simulink model "destilador_10c_sim_dos"  (R2018b)
settings: Solver=VariableStepAuto  StartTime=0.0  StopTime=17290  FixedStep=1  MaxStep=10  RelTol=1e-4  AbsTol=1e-5  EnableMultiTasking=on
InitFcn:
  | %% Condiciones iniciales
  | load('X0_ini_ev') %% 6/7/2018 20:06 cond_inicialx0.m % Cmet=1.5; % V=40; % GA=13; % N=21;
  | 
  | % Parameters
  | Mcp_c=4*50000;
  | Phi_ef=0.99;
  | V_m=20;  %mL volumen
  | Q_loss=0; % watt
  | GLm_0=80;
  | 
  | alpha=0.009;
  | F_fin=150;
  | F_ini=50;
  | 
  | 
  | %% Setting initial condition vector
  | x0_ini2=x0_ini;
  | N=7;
  | x0_ini=zeros(4*N+7,1);
  | x0_ini(1)=x0_ini2(1);
  | x0_ini(2)=x0_ini2(2);
  | x0_ini(3)=x0_ini2(3);
  | for J=1:N
  |   x0_ini(4*J+0)=(x0_ini2(4*J+0+8*(J-1))+x0_ini2(4*J+4+8*(J-1))+x0_ini2(4*J+8+8*(J-1)))/3;
  |   x0_ini(4*J+1)=(x0_ini2(4*J+1+8*(J-1))+x0_ini2(4*J+5+8*(J-1))+x0_ini2(4*J+9+8*(J-1)))/3+0.01;
  |   x0_ini(4*J+2)=(x0_ini2(4*J+2+8*(J-1))+x0_ini2(4*J+6+8*(J-1))+x0_ini2(4*J+10+8*(J-1)))/3;
  |   x0_ini(4*J+3)=(x0_ini2(4*J+3+8*(J-1))+x0_ini2(4*J+7+8*(J-1))+x0_ini2(4*J+11+8*(J-1)))/3;
  | end
  | 
  | b=2;
  | a=1;
  | x_min=[1767.71545621850;0.00799041062661984;3.41060000832915e-05;0.740207193810922;0.00799041062661984;3.41060000832915e-05;352.310691243690;0.740207193810922;0.00799041062661984;3.41060000832915e-05;352.310691243690;0.740207193810922;0.00799041062661984;3.41060000832915e-05;352.310691243690;0.740207193810922;0.00799041062661984;3.41060000832915e-05;352.310691243690;0.740207193810922;0.00799041062661984;3.41060000832915e-05;352.310691243690;0.740207193810922;0.00799041062661984;3.41060000832915e-05;352.310691243690;0.740207193810922;0.00799041062661984;3.41060000832915e-05;352.310691243690;0;0;0;0];
  | x_max=[2018.07587071285;0.624753322576231;0.000637824871562298;1.30537895369255;0.624753322576231;0.000637824871562298;371.461866693347;1.30537895369255;0.624753322576231;0.000637824871562298;371.461866693347;1.30537895369255;0.624753322576231;0.000637824871562298;371.461866693347;1.30537895369255;0.624753322576231;0.000637824871562298;371.461866693347;1.30537895369255;0.624753322576231;0.000637824871562298;371.461866693347;1.30537895369255;0.624753322576231;0.000637824871562298;371.461866693347;1.30537895369255;0.624753322576231;0.000637824871562298;371.461866693347;65.8799169826809;0.143158013086597;184.381691331991;91.0300185684774];
  | x_range=[250.360414494350;0.616762911949612;0.000603718871479006;0.565171759881627;0.616762911949612;0.000603718871479006;19.1511754496572;0.565171759881627;0.616762911949612;0.000603718871479006;19.1511754496572;0.565171759881627;0.616762911949612;0.000603718871479006;19.1511754496572;0.565171759881627;0.616762911949612;0.000603718871479006;19.1511754496572;0.565171759881627;0.616762911949612;0.000603718871479006;19.1511754496572;0.565171759881627;0.616762911949612;0.000603718871479006;19.1511754496572;0.565171759881627;0.616762911949612;0.000603718871479006;19.1511754496572;65.8799169826809;0.143158013086597;184.381691331991;91.0300185684774];
  | x_ss=0.5*(x_max+x_min);
  | 
  | 
  | No=7;  %ecuaciones externas BMyE columna
  | %Ajuste de estados auxiliares
  | x0_ini(4*N+3+1:4*N+No-1)=0;  % estados auxiliares
  | x0_ini(4*N+No)=GLm_0; % estado inicial de GLm
  | 
  | % int_lower_limit=[0 0 0, repmat([0 0 0 273+78],1,N),zeros(1,N-3)]';
  | % int_uper_limit=[5000 1 1, repmat([5 1 1 273+100],1,N),[5000 5000 5000 100]]';
  | 
  | 
  | 
  | 
  | %% Normalization values / mesurements
  | y_ss=76.5;
  | y_max=95;
  | y_min=30;
  | 
  | %% Normalization values / input/disturbances
  | u_ss=[1000 273+25 180];  % [Fr Qb Ti]
  | u_max=[1800 273+50 500];  % [Fr Qb Ti]
  | u_min=[100 273 5];  % [Fr Qb Ti]
values from neighbouring files (symbols this model uses):
  T_fin = dist_exp{i}(end,2)*60    [fcost.m]    (also in fcost_Fr.m; fcost_Fr2.m; fcost_Fr4.m; fcost_Fr5.m)
undefined symbols (not defined in the file or in its folder): Qb_0, Ti_0
libraries: simulink x1, jMPClib x1
(part 2 of 2)

== matlab function destilador_10c_sim_dos/NL Plant Nominal/Implicit Fun ==
  data: x input size=35; w input size=2; f output size=2; u input size=3; p input size=4
function f  = Implicit_fun(x,w,u,p)

Fr     = u(1);   % Flow refrigerant 
Tr     = u(2);   % Temperature refrigerant inlet
Qb     = u(3);   % Heating power boiler

x1c=w(1);  % implicit variable - liquid molar fraction ethanol condenser
Tout=w(2); % implicit variable - Temperature outlet coil condenser

phi_ef = p(1);

% phi_ef=0.701;


N=7;  % stages
No=7; % Aditional stat for output calculation
Ds = 2.047*2.54/100;                                                      % [m]
S = 0.25*pi*Ds^2;                                                   % [m^2]
ap = phi_ef*771; % Nominal, 0.83                                 % [m^2/m^3]                          
l = 0.25;                                                             % [m]
mr = 1933*5/8;                                                         % [g]                         
mrp = mr/l;                                                         % [g/m]
PM_EtOH = 46.07;                                                  % [g/mol]
PM_MetOH = 32.04;                                                 % [g/mol]
PM_H2O = 18.016;                                                  % [g/mol]
CM = 1.130;                                                           % [-]                                   
g = 9.8;                                                          % [m/s^2]
cpr = 0.474;                                                   % [J/(gr*K)]
Ta = 298.45;                                                          % [K]

z = linspace(0,l,N);
dz = z(2)-z(1);

% Luego se leen los estados con el fin de simplificarlo:
Mb = x(1);
x1b = x(2);
x2b = x(3);

M = zeros(1,N);
x1 = zeros(1,N);
x2 = zeros(1,N);
T = zeros(1,N);

for i = 1:N
    M(i) = x(4*i);
    x1(i) = x(4*i+1);
    x2(i) = x(4*i+2);
    T(i) = x(4*i+3);
end

GL_m    = x(4*N+No);  % Estado GL medido

% A continuación se presentan las ecuaciones algebraicas del modelo:
L= flujo_liquido2(M,x1,T,PM_EtOH,PM_H2O,g,ap,S); %vector flujo liquido
h = (55.678*x1+75.425).*T-15208.44*x1-20602.34; %vector de entalpía liquida

% Etapa 5: Presentaci?n de las propiedades del re-hervidor:
y1b = (1220*x1b^3-735.1*x1b^2+1220*x1b+1.498)/(x1b^3+54.93*x1b^2+1538*x1b+113);
Tb = (374.1+5855*x1b)/(1+16.65*x1b+0.1086*x1b^2);
y2b = equil2x(x1b,x2b,Tb);
hb = (55.678*x1b+75.425)*Tb-15208.44*x1b-20602.34;
Hb = 36172.03-2919.83*y1b+(31.461-11.976*y1b)*Tb+(4.063e-4+0.0734*y1b)*Tb^2;
dhbdx1b = 55.678*Tb-15208.44;
dhbdTb = 55.678*x1b+75.425;
dTbdx1b = (5855*(1+16.65*x1b+0.1086*x1b^2)-(374.1+5855*x1b)*(16.65+0.2172*x1b))/((1+16.65*x1b+0.1086*x1b)^2);
Qp = -190.45051+0.027736447*Tb^1.5-0.00069779137*Ta^2+(31705.067/Ta); % [W]
Qbe = Qb-Qp;                                                          % [W]
Vb = (L(1)*((h(1)-hb)+(dhbdx1b+dhbdTb*dTbdx1b)*(x1b-x1(1)))+Qbe)/((dhbdx1b+dhbdTb*dTbdx1b)*(x1b-y1b)+(Hb-hb));

% Etapa 6: C?lculo de las propiedades del vapor que pasa por la columna:
% - Etapa 1:
y1 = zeros(1,N);
y1_1=zeros(1,N);
y1_2=zeros(1,N);

% if T(1) <= 351.89
%     y1(1) = 0.5144798703316682*T(1)^2-362.04116781517121*T(1)+63693.126284857615;
% else if T(1) > 351.89 && T(1) < 362.15
%         y1(1) = -0.00029699079694785408*T(1)^3+0.31993865536139598*T(1)^2-114.90802529355385*T(1)+13759.682820348055;
%     else
%         y1(1) = -0.033707692307692737*T(1)+12.59634076923092;
%     end
% end


if T(1) <= 351.89
    y1(1) = 0.5144798703316682*T(1)^2-362.04116781517121*T(1)+63693.126284857615;
else %if T(1) > 351.89 && T(1) < 362.15
        y1_1(1) = -0.00029699079694785408*T(1)^3+0.31993865536139598*T(1)^2-114.90802529355385*T(1)+13759.682820348055;
%     else
        y1_2(1) = -0.033707692307692737*T(1)+12.59634076923092;
%     end
        sigma=1/(1+exp(-(T(1)-362.15)/1));
        y1(1)=(1-sigma)*y1_1(1)+sigma*y1_2(1);
end


% y1(1)=(1220*x1(1)^3-735.1*x1(1)^2+1220*x1(1)+1.498)/(x1(1)^3+54.93*x1(1)^2+1538*x1(1)+113);
% y1(1)=-3.103366261118440e-07*T(1)^7+ 7.760667779409546e-04*T(1)^6 -0.831728013863949*T(1)^5+ 4.952038647403622e+02*T(1)^4 -1.769012642424244e+05*T(1)^3+3.791596072579136e+07*T(1)^2 -4.514749479837228e+09*T(1)+ 2.303888385771235e+11;
% y1(1)=-1.836023738004047e-07*T(1)^7+ 4.634679433890438e-04*T(1)^6 -0.501379863593959*T(1)^5+ 3.013173444220613e+02*T(1)^4 -1.086463611148553e+05*T(1)^3+ 2.350390640205018e+07*T(1)^2 -2.824717157188236e+09*T(1)+ 1.454841438795462e+11;

    if y1(1)>.8947                                                 %límite azeótropo P atm.
        y1(1)=.8947;
    end

x1i = zeros(1,N);
x1i(1) = 1/(400*y1(1)^4-1299*y1(1)^3+1586*y1(1)^2-865*y1(1)+179.6);

% (PARENTESIS): Se construye un vector de par?metros que es necesario para
% poder llamar al macro transf_masa2:

param = [N PM_EtOH PM_H2O CM ap S g Qb dz 1 mrp cpr Ta]; % Unidades varias.

% Una vez hecho esto se inicializan las variables de flujo molar de vapor
% que sale de cada etapa, coeficientes de transferencia de masa, presi?n de
% vapor del metanol, coeficiente de actividad de ?ste en fase l?quida, u-
% tilizando el modelo de coeficiente de actividad NRTL. Adem?s se definen
% la fracci?n molar de metanol en el vapor y entalp?a de dicha fase,

k13aef = zeros(1,N);
V = zeros(1,N);
k21aef = zeros(1,N);
k23aef = zeros(1,N);
keqaef = zeros(1,N);
P2vap = zeros(1,N);
gama2 = zeros(1,N);
y2 = zeros(1,N);
H = zeros(1,N);

% (FIN DEL PARENTESIS)

Kaef = transf_masa2(x1(1),L(1),T(1),param);
k13aef(1) = Kaef(1,1);
V(1) = ((y1(1)*Vb/dz)+param(10)*S*k13aef(1)*(x1(1)-x1i(1)))/((2*y1(1)-y1b)/dz);
k21aef(1) = Kaef(1,2);
k23aef(1) = Kaef(1,3);
keqaef(1) = (k23aef(1)*k21aef(1)/(x1(1)*k23aef(1)+(1-x1(1))*k21aef(1)));
equil = equilibrio(x1i(1),T(1));
P2vap(1) = equil(1,1);
gama2(1) = equil(1,2);
y2(1) = ((V(1)*y2b/dz)+param(10)*S*keqaef(1)*x2(1))/(((2*V(1)-Vb)/dz)+(param(10)*S*keqaef(1)*101.325/(P2vap(1)*gama2(1))));
H(1) = 36172.03-2919.83*y1(1)+(31.461-11.976*y1(1))*T(1)+(4.063e-4+0.0734*y1(1))*T(1)^2;

% - Etapa 2 a N:
for i = 2:N
    
%     if T(i) <= 351.89
%         y1(i) = 0.5144798703316682*T(i)^2-362.04116781517121*T(i)+63693.126284857615;
%     else if T(i) > 351.89 && T(i) < 362.15
%             y1(i) = -0.00029699079694785408*T(i)^3+0.31993865536139598*T(i)^2-114.90802529355385*T(i)+13759.682820348055;
%         else
%             y1(i) = -0.033707692307692737*T(i)+12.59634076923092;
%         end
%         
%     end
%     
    if T(i) <= 351.89
        y1(i) = 0.5144798703316682*T(i)^2-362.04116781517121*T(i)+63693.126284857615;
    else %if T(i) > 351.89 && T(i) < 362.15
            y1_1(i) = -0.00029699079694785408*T(i)^3+0.31993865536139598*T(i)^2-114.90802529355385*T(i)+13759.682820348055;
%         else
            y1_2(i) = -0.033707692307692737*T(i)+12.59634076923092;
%         end
        sigma=1/(1+exp(-(T(i)-362.15)/1));
        y1(i)=(1-sigma)*y1_1(i)+sigma*y1_2(i);
    end
%     
% y1(i)=(1220*x1(i)^3-735.1*x1(i)^2+1220*x1(i)+1.498)/(x1(i)^3+54.93*x1(i)^2+1538*x1(i)+113);
% y1(i)=-3.103366261118440e-07*T(i)^7+ 7.760667779409546e-04*T(i)^6 -0.831728013863949*T(i)^5+ 4.952038647403622e+02*T(i)^4 -1.769012642424244e+05*T(i)^3+3.791596072579136e+07*T(i)^2 -4.514749479837228e+09*T(i)+ 2.303888385771235e+11;    
% y1(i)=-1.836023738004047e-07*T(i)^7+ 4.634679433890438e-04*T(i)^6 -0.501379863593959*T(i)^5+ 3.013173444220613e+02*T(i)^4 -1.086463611148553e+05*T(i)^3+ 2.350390640205018e+07*T(i)^2 -2.824717157188236e+09*T(i)+ 1.454841438795462e+11;
    if y1(i)>.8947                                                 %límite azeótropo P atm.
        y1(i)=.8947;
    end
    x1i(i) = 1/(400*y1(i)^4-1299*y1(i)^3+1586*y1(i)^2-865*y1(i)+179.6);
    Kaef = transf_masa2(x1(i),L(i),T(i),param);
    k13aef(i) = Kaef(1,1);
    V(i) = ((y1(i)*V(i-1)/dz)+param(10)*S*k13aef(i)*(x1(i)-x1i(i)))/((2*y1(i)-y1(i-1))/dz);
    k21aef(i) = Kaef(1,2);
    k23aef(i) = Kaef(1,3);
    keqaef(i) = (k23aef(i)*k21aef(i)/(x1(i)*k23aef(i)+(1-x1(i))*k21aef(i)));
    equil = equilibrio(x1i(i),T(i));
    P2vap(i) = equil(1,1);
    gama2(i) = equil(1,2);
    y2(i) = ((V(i)*y2(i-1)/dz)+param(10)*S*keqaef(i)*x2(i))/(((2*V(i)-V(i-1))/dz)+(param(10)*S*keqaef(i)*101.325/(P2vap(i)*gama2(i))));
    H(i) = 36172.03-2919.83*y1(i)+(31.461-11.976*y1(i))*T(i)+(4.063e-4+0.0734*y1(i))*T(i)^2;
end

%% Partial Condenser Column-side
% xc Implicit variable

%     T = (369.6-863.6*y1(N)+1049*y1(N)^2)/(1-2.34*y1(N)+2.918*y1(N)^2);                % [K]                 
    Hn = 36172.03-2919.83*y1(N)+(31.461-11.976*y1(N))*T(N)+(4.063e-4+0.0734*y1(N))*T(N)^2; % [J/mol]
    yD = (1220*x1c^3-735.1*x1c^2+1220*x1c+1.498)/(x1c^3+54.93*x1c^2+1538*x1c+113); % [-]
    R = (yD-y1(N))/(y1(N)-x1c);                                              % [-]
    Lc = V(N)/(1+(1/R));                                             % [mol/s]
    Tc = (374.1+5855*x1c)/(1+16.65*x1c+0.1086*x1c^2);                    % [K]
    equil = equilibrio(x1c,Tc);                          % [Unidades varias]                               
    P2vap = equil(1,1);                                             % [kPa]                                                
    gama2 = equil(1,2);                                               % [-]
    x2c = V(N)*y2(N)/(Lc*(1+(P2vap*gama2/(101.325*R))));                    % [-]
    hc = (55.678*x1c+75.425)*Tc-15208.44*x1c-20602.34;              % [J/mol]
    HD = 36172.03-2919.83*yD+(31.461-11.976*yD)*Tc+(4.063e-4+0.0734*yD)*Tc^2; % [J/mol]
    
    Qc_ef = V(N)*Hn-Lc*(hc+(HD/R));                                       % [W]


    
    
%% Partial Condenser Tube-side
% Tout  Implicit variable


T_film = 0.5*(Tr+Tout);                                              % [K]
cp = 0.000008935*T_film^2-0.0054919213*T_film+5.0225997509;   % [kJ/(kg*K)]
mu = exp((-9.108111-(753.33377/T_film)+(410019.22/(T_film^2))));   % [Pa*s]
k = -0.000008072*T_film^2+0.006348737*T_film-0.5649534949;      % [W/(m*K)]
Pr = exp((-8.9216883+0.00000062007495*T_film^2.5+(2915.8766/T_film))); % [-]

% ... y de la temperatura de la pared.

mu_s = exp((-9.108111-(753.33377/Tc)+(410019.22/(Tc^2))));         % [Pa*s]

% Ahora se procede a calcular las condiciones para el número de Nusselt, 
% antes se presentan los parámetros geométricos del serpentín:

As = 157.4776*(0.01^2);                                                  % [m^2]
do = 0.008;                                                           % [m]
di=0.007;
Long = As/(pi*do);                                                       % [m]

rho_def = -0.00295*(Tr)^2+1.45738*(Tr)+824.9622;

m = Fr*rho_def*(1/(60*1000*1000) );                                     % [kg/s]

Re = (4*m)/(pi*di*mu);                                                % [-]
Gz_mod = ((Re*Pr/(Long/do)))^(1/3)*((mu/mu_s))^(0.14);                   % [-]                                           
if (Re < 10000) && (Gz_mod < 2)
    Nu = 3.66;                                                        % [-]
else if (Re < 10000) && (Gz_mod >= 2)
       Nu = 1.86*Gz_mod;                                              % [-]
    else
        Nu = 0.027*Re^(4/5)*Pr^(1/3)*(mu/mu_s)^(0.14);                % [-]
    end
end

% Tras esto se calcula el coeficiente de transferencia de calor para el
% flujo refrigerante:

h_conv = k*Nu/do;                                                  % [W/(m^2*K)]

% Finalmente se calcula el largo del serpentín de dos formas independientes
% y se realiza la comparación entre ellos y la salida:

dTml = (Tout-Tr)/log((Tc-Tr)/(Tc-Tout))    ;                       % [K]
% dTml =(Tout*Tr*(Tr+Tc)/2)^(1/3);
Qc_I = h_conv*As*dTml;                                                     % [W]

 
cp_def = 0.000008935*(0.5*(Tr+Tout))^2-0.0054919213*(0.5*(Tr+Tout))+5.0225997509; % [kJ/(kg*K)]


Qc= Fr*(1/(60*1000)) * cp_def * (Tout-Tr) * rho_def;
    
% 
% destil = destilado(V(N),y1(N),y2(N),Lc,x1c,x2c,PM_EtOH,PM_H2O);
% GL=destil(1,1);
% Dvol=destil(1,2);
%     salida = [GL Dvol D_EtOH D_MEtOH D_H2O];  


f=zeros(2,1);
f(1)= (Qc-Qc_ef);  % Implicit equation 1
f(2)= (Qc-Qc_I);  % Implicit equation 2

== matlab function destilador_10c_sim_dos/NL Plant Nominal/ODE Distiller ==
  data: x input size=35; w input size=2; x_dot output size=35; u input size=3; y output size=12; p input size=4; x0 input size=35
function [x_dot,y] = ODE_Distiller(x,w,u,p,x0)
% Fr     = u(1);   % Flow refrigerant 
% Tr     = u(2);   % Temperature refrigerant inlet
Qb     = u(3);   % Heating power boiler

x1c=w(1);  % implicit variable - liquid molar fraction ethanol condenser
% Tout=w(2); % implicit variable - Temperature outlet coil condenser

phi_ef = p(1);
Mcp_c=p(2);
Q_loss=p(4);

N=7;  % stages
No=7; % Aditional stat for output calculation
Ds = 2.047*2.54/100;                                                      % [m]
S = 0.25*pi*Ds^2;                                                   % [m^2]
ap = phi_ef*771; % Nominal, 0.83                                 % [m^2/m^3]                          
l = 0.25;                                                             % [m]
mr = 1933*5/8;                                                         % [g]                         
mrp = mr/l;                                                         % [g/m]
PM_EtOH = 46.07;                                                  % [g/mol]
PM_MetOH = 32.04;                                                 % [g/mol]
PM_H2O = 18.016;                                                  % [g/mol]
CM = 1.130;                                                           % [-]                                   
g = 9.8;                                                          % [m/s^2]
cpr = 0.474;                                                   % [J/(gr*K)]
Ta = 298.45;                                                          % [K]

z = linspace(0,l,N);
dz = z(2)-z(1);

% Luego se leen los estados con el fin de simplificarlo:
Mb = x(1);
x1b = x(2);
x2b = x(3);

M =x(4+0:4:4*N+0);
x1=x(4+1:4:4*N+1);
x2=x(4+2:4:4*N+2);
T =x(4+3:4:4*N+3);

GL_m    = x(4*N+No);  % Estado GL medido

% A continuación se presentan las ecuaciones algebraicas del modelo:
L= flujo_liquido2(M,x1,T,PM_EtOH,PM_H2O,g,ap,S); %vector flujo liquido
h = (55.678*x1+75.425).*T-15208.44*x1-20602.34; %vector de entalpía liquida

% Etapa 5: Presentaci?n de las propiedades del re-hervidor:
coef_num_y_eq=[1220 -735.1 1220 1.498];
coef_den_y_eq=[1 54.93 1538 113];
y1b = polyval(coef_num_y_eq,x1b)/polyval(coef_den_y_eq,x1b);

Tb = (374.1+5855*x1b)/(1+16.65*x1b+0.1086*x1b^2);
y2b = equil2x(x1b,x2b,Tb);
hb = (55.678*x1b+75.425)*Tb-15208.44*x1b-20602.34;
Hb = 36172.03-2919.83*y1b+(31.461-11.976*y1b)*Tb+(4.063e-4+0.0734*y1b)*Tb^2;
dhbdx1b = 55.678*Tb-15208.44;
dhbdTb = 55.678*x1b+75.425;
dTbdx1b = (5855*(1+16.65*x1b+0.1086*x1b^2)-(374.1+5855*x1b)*(16.65+0.2172*x1b))/((1+16.65*x1b+0.1086*x1b)^2);
Qp = -190.45051+0.027736447*Tb^1.5-0.00069779137*Ta^2+(31705.067/Ta); % [W]
Qbe = Qb-Qp;                                                          % [W]
Vb = (L(1)*((h(1)-hb)+(dhbdx1b+dhbdTb*dTbdx1b)*(x1b-x1(1)))+Qbe)/((dhbdx1b+dhbdTb*dTbdx1b)*(x1b-y1b)+(Hb-hb));



y1_1 = -0.00029699079694785408*T.^3+0.31993865536139598*T.^2-114.90802529355385*T+13759.682820348055;
y1_2 = -0.033707692307692737*T+12.59634076923092;
sigma=1./(1+exp(-(T-362.15)/1));
y1=(1-sigma).*y1_1+sigma.*y1_2;


x1i = 1./(400*y1.^4-1299*y1.^3+1586*y1.^2-865*y1+179.6);

param = [N PM_EtOH PM_H2O CM ap S g Qb dz 1 mrp cpr Ta]; % Unidades varias.

% Una vez hecho esto se inicializan las variables de flujo molar de vapor
% que sale de cada etapa, coeficientes de transferencia de masa, presi?n de
% vapor del metanol, coeficiente de actividad de ?ste en fase l?quida, u-
% tilizando el modelo de coeficiente de actividad NRTL. Adem?s se definen
% la fracci?n molar de metanol en el vapor y entalp?a de dicha fase,

k13aef = zeros(1,N);
V = zeros(1,N);
k21aef = zeros(1,N);
k23aef = zeros(1,N);
keqaef = zeros(1,N);
P2vap = zeros(1,N);
gama2 = zeros(1,N);
y2 = zeros(1,N);
H = zeros(1,N);

% (FIN DEL PARENTESIS)

Kaef = transf_masa2(x1(1),L(1),T(1),param);
k13aef(1) = Kaef(1,1);
V(1) = ((y1(1)*Vb/dz)+param(10)*S*k13aef(1)*(x1(1)-x1i(1)))/((2*y1(1)-y1b)/dz);
k21aef(1) = Kaef(1,2);
k23aef(1) = Kaef(1,3);
keqaef(1) = (k23aef(1)*k21aef(1)/(x1(1)*k23aef(1)+(1-x1(1))*k21aef(1)));
equil = equilibrio(x1i(1),T(1));
P2vap(1) = equil(1,1);
gama2(1) = equil(1,2);
y2(1) = ((V(1)*y2b/dz)+param(10)*S*keqaef(1)*x2(1))/(((2*V(1)-Vb)/dz)+(param(10)*S*keqaef(1)*101.325/(P2vap(1)*gama2(1))));
H(1) = 36172.03-2919.83*y1(1)+(31.461-11.976*y1(1))*T(1)+(4.063e-4+0.0734*y1(1))*T(1)^2;


for i = 2:N
    Kaef = transf_masa2(x1(i),L(i),T(i),param);
    k13aef(i) = Kaef(1,1);
    V(i) = ((y1(i)*V(i-1)/dz)+param(10)*S*k13aef(i)*(x1(i)-x1i(i)))/((2*y1(i)-y1(i-1))/dz);
    k21aef(i) = Kaef(1,2);
    k23aef(i) = Kaef(1,3);
    keqaef(i) = (k23aef(i)*k21aef(i)/(x1(i)*k23aef(i)+(1-x1(i))*k21aef(i)));
    equil = equilibrio(x1i(i),T(i));
    P2vap(i) = equil(1,1);
    gama2(i) = equil(1,2);
    y2(i) = ((V(i)*y2(i-1)/dz)+param(10)*S*keqaef(i)*x2(i))/(((2*V(i)-V(i-1))/dz)+(param(10)*S*keqaef(i)*101.325/(P2vap(i)*gama2(i))));
    H(i) = 36172.03-2919.83*y1(i)+(31.461-11.976*y1(i))*T(i)+(4.063e-4+0.0734*y1(i))*T(i)^2;
end

    yD = polyval(coef_num_y_eq,x1c)/polyval(coef_den_y_eq,x1c);
    R = (yD-y1(N))/(y1(N)-x1c);                                              % [-]
    Lc = V(N)/(1+(1/R));                                             % [mol/s]
    Tc = (374.1+5855*x1c)/(1+16.65*x1c+0.1086*x1c^2);                    % [K]
    equil = equilibrio(x1c,Tc);                          % [Unidades varias]                               
    P2vap = equil(1,1);                                             % [kPa]                                                
    gama2 = equil(1,2);                                               % [-]
    x2c = V(N)*y2(N)/(Lc*(1+(P2vap*gama2/(101.325*R))));                    % [-]
    hc = (55.678*x1c+75.425)*Tc-15208.44*x1c-20602.34;              % [J/mol]

% Finalmente se presentan las ecuaciones diferenciales del modelo:
x_dot=zeros(4*N+No,1);

x_dot(1) = L(1)-Vb;
x_dot(2) = (1/Mb)*(L(1)*(x1(1)-x1b)-Vb*(y1b-x1b));
x_dot(3) = (1/Mb)*(L(1)*(x2(1)-x2b)-Vb*(y2b-x2b));
x_dot(4) = ((L(2)-L(1))/dz)+((Vb-V(1))/dz);
x_dot(5) = (1/M(1))*(L(1)*((x1(2)-x1(1))/dz)+V(1)*((y1b-y1(1))/dz)+(x1(1)-y1(1))*((V(1)-Vb)/dz));
x_dot(6) = (1/M(1))*(L(1)*((x2(2)-x2(1))/dz)+V(1)*((y2b-y2(1))/dz)+(x2(1)-y2(1))*((V(1)-Vb)/dz));
x_dot(7) = ((Mcp_c+mrp*cpr+M(1)*(55.678*x1(1)+75.425))^-1)*(-Q_loss/dz+L(1)*((h(2)-h(1))/dz)+V(1)*((Hb-H(1))/dz)+(h(1)-H(1))*((V(1)-Vb)/dz)-(55.678*T(1)-15208.44)*(L(1)*((x1(2)-x1(1))/dz)+V(1)*((y1b-y1(1))/dz)+(x1(1)-y1(1))*((V(1)-Vb)/dz)));
for i = 2:(N-1)
    x_dot(4*i) = ((L(i+1)-L(i))/dz)+((V(i-1)-V(i))/dz);
    x_dot(4*i+1) = (1/M(i))*(L(i)*((x1(i+1)-x1(i))/dz)+V(i)*((y1(i-1)-y1(i))/dz)+(x1(i)-y1(i))*((V(i)-V(i-1))/dz));
    x_dot(4*i+2) = (1/M(i))*(L(i)*((x2(i+1)-x2(i))/dz)+V(i)*((y2(i-1)-y2(i))/dz)+(x2(i)-y2(i))*((V(i)-V(i-1))/dz));
    x_dot(4*i+3) = ((Mcp_c+mrp*cpr+M(i)*(55.678*x1(i)+75.425))^-1)*(-Q_loss/dz+L(i)*((h(i+1)-h(i))/dz)+V(i)*((H(i-1)-H(i))/dz)+(h(i)-H(i))*((V(i)-V(i-1))/dz)-(55.678*T(i)-15208.44)*(L(i)*((x1(i+1)-x1(i))/dz)+V(i)*((y1(i-1)-y1(i))/dz)+(x1(i)-y1(i))*((V(i)-V(i-1))/dz)));
end
x_dot(4*N) = ((Lc-L(N))/dz)+((V(N-1)-V(N))/dz);
x_dot(4*N+1) = (1/M(N))*(L(N)*((x1c-x1(N))/dz)+V(N)*((y1(N-1)-y1(N))/dz)+(x1(N)-y1(N))*((V(N)-V(N-1))/dz));
x_dot(4*N+2) = (1/M(N))*(L(N)*((x2c-x2(N))/dz)+V(N)*((y2(N-1)-y2(N))/dz)+(x2(N)-y2(N))*((V(N)-V(N-1))/dz));
x_dot(4*N+3) = ((Mcp_c+mrp*cpr+M(N)*(55.678*x1(N)+75.425))^-1)*(-Q_loss/dz+L(N)*((hc-h(N))/dz)+V(N)*((H(N-1)-H(N))/dz)+(h(N)-H(N))*((V(N)-V(N-1))/dz)-(55.678*T(N)-15208.44)*(L(N)*((x1c-x1(N))/dz)+V(N)*((y1(N-1)-y1(N))/dz)+(x1(N)-y1(N))*((V(N)-V(N-1))/dz)));

% Se procede a calcular el volumen de destilado que es retirado del siste-
% ma:
destil = destilado(V(N),y1(N),y2(N),Lc,x1c,x2c,PM_EtOH,PM_H2O);
GL=destil(1,1);
Dvol=destil(1,2);
%     salida = [GL Dvol D_EtOH D_MEtOH D_H2O];  

x_dot(4*N+4) = destil(1,3);  %33  D_EtOH
x_dot(4*N+5) = destil(1,4);  %34  D_MEtOH
x_dot(4*N+6) = destil(1,5);  %34  D_H2O
x_dot(4*N+7)= (GL-GL_m)/(7.35/Dvol);    %40 Eq. dif sensor, cte tiempo: V/Dvol (seg)

N_et=x(4*N+4);
N_met=x(4*N+5);
N_w=x(4*N+6);

%% Output variables calculation
x1_ac=N_et/(N_et+N_met+N_w) ; % Ethanol mole fraction destilate drum
x2_ac=N_met/(N_et+N_met+N_w); % Methanol mole fraction distilate drum
dens_ac = densidad(x1_ac,293.15,PM_EtOH,PM_H2O); 
rho_1ac=dens_ac(1,2); % pure alcohol density in destialte drum
rho_13ac=dens_ac(1,3); % solution density in destialte drum
Mt=N_et*PM_EtOH+N_met*PM_MetOH+N_w*PM_H2O;
rho_methanol=0.789; % Density of pure methanol 20°C
Cmet=x2_ac*(1/rho_methanol)*1000;
GL_ac=x1_ac*(1/rho_1ac)*100/(1/rho_13ac);
Rec_eth=N_et*100/(x0(1)*x0(2));
Rec_met=N_met*100/(x0(1)*x0(3));

y=zeros(12,1);
y(1) = GL_m;   %35  GL
y(2)=GL;
y(3)=GL_ac;  %mL/s  Volumetric flow
y(4) =Tc;    %36  Tc
y(5) =Tb;    %37  
y(6) =x1c;   %38
y(7) =x2c;    %39
y(8)=Cmet;   %g/L a.a.
y(9)=Rec_eth;   %Ethanol molar flow mol/s
y(10)=Rec_met;   %Methanol molar flow mol/s
y(11)=Mt*rho_13ac/1000 ; % Destilate volumen  L
y(12)=Dvol; %mL/min Flow distillate

== matlab function destilador_10c_sim_dos/NL Plant Nominal1/Implicit Fun ==
  data: x input size=35; w input size=2; f output size=2; u input size=3; p input size=4
function f  = Implicit_fun(x,w,u,p)

Fr     = u(1);   % Flow refrigerant 
Tr     = u(2);   % Temperature refrigerant inlet
Qb     = u(3);   % Heating power boiler

x1c=w(1);  % implicit variable - liquid molar fraction ethanol condenser
Tout=w(2); % implicit variable - Temperature outlet coil condenser

phi_ef = p(1);

% phi_ef=0.701;


N=7;  % stages
No=7; % Aditional stat for output calculation
Ds = 2.047*2.54/100;                                                      % [m]
S = 0.25*pi*Ds^2;                                                   % [m^2]
ap = phi_ef*771; % Nominal, 0.83                                 % [m^2/m^3]                          
l = 0.25;                                                             % [m]
mr = 1933*5/8;                                                         % [g]                         
mrp = mr/l;                                                         % [g/m]
PM_EtOH = 46.07;                                                  % [g/mol]
PM_MetOH = 32.04;                                                 % [g/mol]
PM_H2O = 18.016;                                                  % [g/mol]
CM = 1.130;                                                           % [-]                                   
g = 9.8;                                                          % [m/s^2]
cpr = 0.474;                                                   % [J/(gr*K)]
Ta = 298.45;                                                          % [K]

z = linspace(0,l,N);
dz = z(2)-z(1);

% Luego se leen los estados con el fin de simplificarlo:
Mb = x(1);
x1b = x(2);
x2b = x(3);

M = zeros(1,N);
x1 = zeros(1,N);
x2 = zeros(1,N);
T = zeros(1,N);

for i = 1:N
    M(i) = x(4*i);
    x1(i) = x(4*i+1);
    x2(i) = x(4*i+2);
    T(i) = x(4*i+3);
end

GL_m    = x(4*N+No);  % Estado GL medido

% A continuación se presentan las ecuaciones algebraicas del modelo:
L= flujo_liquido2(M,x1,T,PM_EtOH,PM_H2O,g,ap,S); %vector flujo liquido
h = (55.678*x1+75.425).*T-15208.44*x1-20602.34; %vector de entalpía liquida

% Etapa 5: Presentaci?n de las propiedades del re-hervidor:
y1b = (1220*x1b^3-735.1*x1b^2+1220*x1b+1.498)/(x1b^3+54.93*x1b^2+1538*x1b+113);
Tb = (374.1+5855*x1b)/(1+16.65*x1b+0.1086*x1b^2);
y2b = equil2x(x1b,x2b,Tb);
hb = (55.678*x1b+75.425)*Tb-15208.44*x1b-20602.34;
Hb = 36172.03-2919.83*y1b+(31.461-11.976*y1b)*Tb+(4.063e-4+0.0734*y1b)*Tb^2;
dhbdx1b = 55.678*Tb-15208.44;
dhbdTb = 55.678*x1b+75.425;
dTbdx1b = (5855*(1+16.65*x1b+0.1086*x1b^2)-(374.1+5855*x1b)*(16.65+0.2172*x1b))/((1+16.65*x1b+0.1086*x1b)^2);
Qp = -190.45051+0.027736447*Tb^1.5-0.00069779137*Ta^2+(31705.067/Ta); % [W]
Qbe = Qb-Qp;                                                          % [W]
Vb = (L(1)*((h(1)-hb)+(dhbdx1b+dhbdTb*dTbdx1b)*(x1b-x1(1)))+Qbe)/((dhbdx1b+dhbdTb*dTbdx1b)*(x1b-y1b)+(Hb-hb));

% Etapa 6: C?lculo de las propiedades del vapor que pasa por la columna:
% - Etapa 1:
y1 = zeros(1,N);
y1_1=zeros(1,N);
y1_2=zeros(1,N);

% if T(1) <= 351.89
%     y1(1) = 0.5144798703316682*T(1)^2-362.04116781517121*T(1)+63693.126284857615;
% else if T(1) > 351.89 && T(1) < 362.15
%         y1(1) = -0.00029699079694785408*T(1)^3+0.31993865536139598*T(1)^2-114.90802529355385*T(1)+13759.682820348055;
%     else
%         y1(1) = -0.033707692307692737*T(1)+12.59634076923092;
%     end
% end


if T(1) <= 351.89
    y1(1) = 0.5144798703316682*T(1)^2-362.04116781517121*T(1)+63693.126284857615;
else %if T(1) > 351.89 && T(1) < 362.15
        y1_1(1) = -0.00029699079694785408*T(1)^3+0.31993865536139598*T(1)^2-114.90802529355385*T(1)+13759.682820348055;
%     else
        y1_2(1) = -0.033707692307692737*T(1)+12.59634076923092;
%     end
        sigma=1/(1+exp(-(T(1)-362.15)/1));
        y1(1)=(1-sigma)*y1_1(1)+sigma*y1_2(1);
end


% y1(1)=(1220*x1(1)^3-735.1*x1(1)^2+1220*x1(1)+1.498)/(x1(1)^3+54.93*x1(1)^2+1538*x1(1)+113);
% y1(1)=-3.103366261118440e-07*T(1)^7+ 7.760667779409546e-04*T(1)^6 -0.831728013863949*T(1)^5+ 4.952038647403622e+02*T(1)^4 -1.769012642424244e+05*T(1)^3+3.791596072579136e+07*T(1)^2 -4.514749479837228e+09*T(1)+ 2.303888385771235e+11;
% y1(1)=-1.836023738004047e-07*T(1)^7+ 4.634679433890438e-04*T(1)^6 -0.501379863593959*T(1)^5+ 3.013173444220613e+02*T(1)^4 -1.086463611148553e+05*T(1)^3+ 2.350390640205018e+07*T(1)^2 -2.824717157188236e+09*T(1)+ 1.454841438795462e+11;

    if y1(1)>.8947                                                 %límite azeótropo P atm.
        y1(1)=.8947;
    end

x1i = zeros(1,N);
x1i(1) = 1/(400*y1(1)^4-1299*y1(1)^3+1586*y1(1)^2-865*y1(1)+179.6);

% (PARENTESIS): Se construye un vector de par?metros que es necesario para
% poder llamar al macro transf_masa2:

param = [N PM_EtOH PM_H2O CM ap S g Qb dz 1 mrp cpr Ta]; % Unidades varias.

% Una vez hecho esto se inicializan las variables de flujo molar de vapor
% que sale de cada etapa, coeficientes de transferencia de masa, presi?n de
% vapor del metanol, coeficiente de actividad de ?ste en fase l?quida, u-
% tilizando el modelo de coeficiente de actividad NRTL. Adem?s se definen
% la fracci?n molar de metanol en el vapor y entalp?a de dicha fase,

k13aef = zeros(1,N);
V = zeros(1,N);
k21aef = zeros(1,N);
k23aef = zeros(1,N);
keqaef = zeros(1,N);
P2vap = zeros(1,N);
gama2 = zeros(1,N);
y2 = zeros(1,N);
H = zeros(1,N);

% (FIN DEL PARENTESIS)

Kaef = transf_masa2(x1(1),L(1),T(1),param);
k13aef(1) = Kaef(1,1);
V(1) = ((y1(1)*Vb/dz)+param(10)*S*k13aef(1)*(x1(1)-x1i(1)))/((2*y1(1)-y1b)/dz);
k21aef(1) = Kaef(1,2);
k23aef(1) = Kaef(1,3);
keqaef(1) = (k23aef(1)*k21aef(1)/(x1(1)*k23aef(1)+(1-x1(1))*k21aef(1)));
equil = equilibrio(x1i(1),T(1));
P2vap(1) = equil(1,1);
gama2(1) = equil(1,2);
y2(1) = ((V(1)*y2b/dz)+param(10)*S*keqaef(1)*x2(1))/(((2*V(1)-Vb)/dz)+(param(10)*S*keqaef(1)*101.325/(P2vap(1)*gama2(1))));
H(1) = 36172.03-2919.83*y1(1)+(31.461-11.976*y1(1))*T(1)+(4.063e-4+0.0734*y1(1))*T(1)^2;

% - Etapa 2 a N:
for i = 2:N
    
%     if T(i) <= 351.89
%         y1(i) = 0.5144798703316682*T(i)^2-362.04116781517121*T(i)+63693.126284857615;
%     else if T(i) > 351.89 && T(i) < 362.15
%             y1(i) = -0.00029699079694785408*T(i)^3+0.31993865536139598*T(i)^2-114.90802529355385*T(i)+13759.682820348055;
%         else
%             y1(i) = -0.033707692307692737*T(i)+12.59634076923092;
%         end
%         
%     end
%     
    if T(i) <= 351.89
        y1(i) = 0.5144798703316682*T(i)^2-362.04116781517121*T(i)+63693.126284857615;
    else %if T(i) > 351.89 && T(i) < 362.15
            y1_1(i) = -0.00029699079694785408*T(i)^3+0.31993865536139598*T(i)^2-114.90802529355385*T(i)+13759.682820348055;
%         else
            y1_2(i) = -0.033707692307692737*T(i)+12.59634076923092;
%         end
        sigma=1/(1+exp(-(T(i)-362.15)/1));
        y1(i)=(1-sigma)*y1_1(i)+sigma*y1_2(i);
    end
%     
% y1(i)=(1220*x1(i)^3-735.1*x1(i)^2+1220*x1(i)+1.498)/(x1(i)^3+54.93*x1(i)^2+1538*x1(i)+113);
% y1(i)=-3.103366261118440e-07*T(i)^7+ 7.760667779409546e-04*T(i)^6 -0.831728013863949*T(i)^5+ 4.952038647403622e+02*T(i)^4 -1.769012642424244e+05*T(i)^3+3.791596072579136e+07*T(i)^2 -4.514749479837228e+09*T(i)+ 2.303888385771235e+11;    
% y1(i)=-1.836023738004047e-07*T(i)^7+ 4.634679433890438e-04*T(i)^6 -0.501379863593959*T(i)^5+ 3.013173444220613e+02*T(i)^4 -1.086463611148553e+05*T(i)^3+ 2.350390640205018e+07*T(i)^2 -2.824717157188236e+09*T(i)+ 1.454841438795462e+11;
    if y1(i)>.8947                                                 %límite azeótropo P atm.
        y1(i)=.8947;
    end
    x1i(i) = 1/(400*y1(i)^4-1299*y1(i)^3+1586*y1(i)^2-865*y1(i)+179.6);
    Kaef = transf_masa2(x1(i),L(i),T(i),param);
    k13aef(i) = Kaef(1,1);
    V(i) = ((y1(i)*V(i-1)/dz)+param(10)*S*k13aef(i)*(x1(i)-x1i(i)))/((2*y1(i)-y1(i-1))/dz);
    k21aef(i) = Kaef(1,2);
    k23aef(i) = Kaef(1,3);
    keqaef(i) = (k23aef(i)*k21aef(i)/(x1(i)*k23aef(i)+(1-x1(i))*k21aef(i)));
    equil = equilibrio(x1i(i),T(i));
    P2vap(i) = equil(1,1);
    gama2(i) = equil(1,2);
    y2(i) = ((V(i)*y2(i-1)/dz)+param(10)*S*keqaef(i)*x2(i))/(((2*V(i)-V(i-1))/dz)+(param(10)*S*keqaef(i)*101.325/(P2vap(i)*gama2(i))));
    H(i) = 36172.03-2919.83*y1(i)+(31.461-11.976*y1(i))*T(i)+(4.063e-4+0.0734*y1(i))*T(i)^2;
end

%% Partial Condenser Column-side
% xc Implicit variable

%     T = (369.6-863.6*y1(N)+1049*y1(N)^2)/(1-2.34*y1(N)+2.918*y1(N)^2);                % [K]                 
    Hn = 36172.03-2919.83*y1(N)+(31.461-11.976*y1(N))*T(N)+(4.063e-4+0.0734*y1(N))*T(N)^2; % [J/mol]
    yD = (1220*x1c^3-735.1*x1c^2+1220*x1c+1.498)/(x1c^3+54.93*x1c^2+1538*x1c+113); % [-]
    R = (yD-y1(N))/(y1(N)-x1c);                                              % [-]
    Lc = V(N)/(1+(1/R));                                             % [mol/s]
    Tc = (374.1+5855*x1c)/(1+16.65*x1c+0.1086*x1c^2);                    % [K]
    equil = equilibrio(x1c,Tc);                          % [Unidades varias]                               
    P2vap = equil(1,1);                                             % [kPa]                                                
    gama2 = equil(1,2);                                               % [-]
    x2c = V(N)*y2(N)/(Lc*(1+(P2vap*gama2/(101.325*R))));                    % [-]
    hc = (55.678*x1c+75.425)*Tc-15208.44*x1c-20602.34;              % [J/mol]
    HD = 36172.03-2919.83*yD+(31.461-11.976*yD)*Tc+(4.063e-4+0.0734*yD)*Tc^2; % [J/mol]
    
    Qc_ef = V(N)*Hn-Lc*(hc+(HD/R));                                       % [W]


    
    
%% Partial Condenser Tube-side
% Tout  Implicit variable


T_film = 0.5*(Tr+Tout);                                              % [K]
cp = 0.000008935*T_film^2-0.0054919213*T_film+5.0225997509;   % [kJ/(kg*K)]
mu = exp((-9.108111-(753.33377/T_film)+(410019.22/(T_film^2))));   % [Pa*s]
k = -0.000008072*T_film^2+0.006348737*T_film-0.5649534949;      % [W/(m*K)]
Pr = exp((-8.9216883+0.00000062007495*T_film^2.5+(2915.8766/T_film))); % [-]

% ... y de la temperatura de la pared.

mu_s = exp((-9.108111-(753.33377/Tc)+(410019.22/(Tc^2))));         % [Pa*s]

% Ahora se procede a calcular las condiciones para el número de Nusselt, 
% antes se presentan los parámetros geométricos del serpentín:

As = 157.4776*(0.01^2);                                                  % [m^2]
do = 0.008;                                                           % [m]
di=0.007;
Long = As/(pi*do);                                                       % [m]

rho_def = -0.00295*(Tr)^2+1.45738*(Tr)+824.9622;

m = Fr*rho_def*(1/(60*1000*1000) );                                     % [kg/s]

Re = (4*m)/(pi*di*mu);                                                % [-]
Gz_mod = ((Re*Pr/(Long/do)))^(1/3)*((mu/mu_s))^(0.14);                   % [-]                                           
if (Re < 10000) && (Gz_mod < 2)
    Nu = 3.66;                                                        % [-]
else if (Re < 10000) && (Gz_mod >= 2)
       Nu = 1.86*Gz_mod;                                              % [-]
    else
        Nu = 0.027*Re^(4/5)*Pr^(1/3)*(mu/mu_s)^(0.14);                % [-]
    end
end

% Tras esto se calcula el coeficiente de transferencia de calor para el
% flujo refrigerante:

h_conv = k*Nu/do;                                                  % [W/(m^2*K)]

% Finalmente se calcula el largo del serpentín de dos formas independientes
% y se realiza la comparación entre ellos y la salida:

dTml = (Tout-Tr)/log((Tc-Tr)/(Tc-Tout))    ;                       % [K]
% dTml =(Tout*Tr*(Tr+Tc)/2)^(1/3);
Qc_I = h_conv*As*dTml;                                                     % [W]

 
cp_def = 0.000008935*(0.5*(Tr+Tout))^2-0.0054919213*(0.5*(Tr+Tout))+5.0225997509; % [kJ/(kg*K)]


Qc= Fr*(1/(60*1000)) * cp_def * (Tout-Tr) * rho_def;
    
% 
% destil = destilado(V(N),y1(N),y2(N),Lc,x1c,x2c,PM_EtOH,PM_H2O);
% GL=destil(1,1);
% Dvol=destil(1,2);
%     salida = [GL Dvol D_EtOH D_MEtOH D_H2O];  


f=zeros(2,1);
f(1)= (Qc-Qc_ef);  % Implicit equation 1
f(2)= (Qc-Qc_I);  % Implicit equation 2

== matlab function destilador_10c_sim_dos/NL Plant Nominal1/ODE Distiller ==
  data: x input size=35; w input size=2; x_dot output size=35; u input size=3; y output size=12; p input size=4; x0 input size=35
function [x_dot,y] = ODE_Distiller(x,w,u,p,x0)
% Fr     = u(1);   % Flow refrigerant 
% Tr     = u(2);   % Temperature refrigerant inlet
Qb     = u(3);   % Heating power boiler

x1c=w(1);  % implicit variable - liquid molar fraction ethanol condenser
% Tout=w(2); % implicit variable - Temperature outlet coil condenser

phi_ef = p(1);
Mcp_c=p(2);
Q_loss=p(4);

N=7;  % stages
No=7; % Aditional stat for output calculation
Ds = 2.047*2.54/100;                                                      % [m]
S = 0.25*pi*Ds^2;                                                   % [m^2]
ap = phi_ef*771; % Nominal, 0.83                                 % [m^2/m^3]                          
l = 0.25;                                                             % [m]
mr = 1933*5/8;                                                         % [g]                         
mrp = mr/l;                                                         % [g/m]
PM_EtOH = 46.07;                                                  % [g/mol]
PM_MetOH = 32.04;                                                 % [g/mol]
PM_H2O = 18.016;                                                  % [g/mol]
CM = 1.130;                                                           % [-]                                   
g = 9.8;                                                          % [m/s^2]
cpr = 0.474;                                                   % [J/(gr*K)]
Ta = 298.45;                                                          % [K]

z = linspace(0,l,N);
dz = z(2)-z(1);

% Luego se leen los estados con el fin de simplificarlo:
Mb = x(1);
x1b = x(2);
x2b = x(3);

M =x(4+0:4:4*N+0);
x1=x(4+1:4:4*N+1);
x2=x(4+2:4:4*N+2);
T =x(4+3:4:4*N+3);

GL_m    = x(4*N+No);  % Estado GL medido

% A continuación se presentan las ecuaciones algebraicas del modelo:
L= flujo_liquido2(M,x1,T,PM_EtOH,PM_H2O,g,ap,S); %vector flujo liquido
h = (55.678*x1+75.425).*T-15208.44*x1-20602.34; %vector de entalpía liquida

% Etapa 5: Presentaci?n de las propiedades del re-hervidor:
coef_num_y_eq=[1220 -735.1 1220 1.498];
coef_den_y_eq=[1 54.93 1538 113];
y1b = polyval(coef_num_y_eq,x1b)/polyval(coef_den_y_eq,x1b);

Tb = (374.1+5855*x1b)/(1+16.65*x1b+0.1086*x1b^2);
y2b = equil2x(x1b,x2b,Tb);
hb = (55.678*x1b+75.425)*Tb-15208.44*x1b-20602.34;
Hb = 36172.03-2919.83*y1b+(31.461-11.976*y1b)*Tb+(4.063e-4+0.0734*y1b)*Tb^2;
dhbdx1b = 55.678*Tb-15208.44;
dhbdTb = 55.678*x1b+75.425;
dTbdx1b = (5855*(1+16.65*x1b+0.1086*x1b^2)-(374.1+5855*x1b)*(16.65+0.2172*x1b))/((1+16.65*x1b+0.1086*x1b)^2);
Qp = -190.45051+0.027736447*Tb^1.5-0.00069779137*Ta^2+(31705.067/Ta); % [W]
Qbe = Qb-Qp;                                                          % [W]
Vb = (L(1)*((h(1)-hb)+(dhbdx1b+dhbdTb*dTbdx1b)*(x1b-x1(1)))+Qbe)/((dhbdx1b+dhbdTb*dTbdx1b)*(x1b-y1b)+(Hb-hb));



y1_1 = -0.00029699079694785408*T.^3+0.31993865536139598*T.^2-114.90802529355385*T+13759.682820348055;
y1_2 = -0.033707692307692737*T+12.59634076923092;
sigma=1./(1+exp(-(T-362.15)/1));
y1=(1-sigma).*y1_1+sigma.*y1_2;


x1i = 1./(400*y1.^4-1299*y1.^3+1586*y1.^2-865*y1+179.6);

param = [N PM_EtOH PM_H2O CM ap S g Qb dz 1 mrp cpr Ta]; % Unidades varias.

% Una vez hecho esto se inicializan las variables de flujo molar de vapor
% que sale de cada etapa, coeficientes de transferencia de masa, presi?n de
% vapor del metanol, coeficiente de actividad de ?ste en fase l?quida, u-
% tilizando el modelo de coeficiente de actividad NRTL. Adem?s se definen
% la fracci?n molar de metanol en el vapor y entalp?a de dicha fase,

k13aef = zeros(1,N);
V = zeros(1,N);
k21aef = zeros(1,N);
k23aef = zeros(1,N);
keqaef = zeros(1,N);
P2vap = zeros(1,N);
gama2 = zeros(1,N);
y2 = zeros(1,N);
H = zeros(1,N);

% (FIN DEL PARENTESIS)

Kaef = transf_masa2(x1(1),L(1),T(1),param);
k13aef(1) = Kaef(1,1);
V(1) = ((y1(1)*Vb/dz)+param(10)*S*k13aef(1)*(x1(1)-x1i(1)))/((2*y1(1)-y1b)/dz);
k21aef(1) = Kaef(1,2);
k23aef(1) = Kaef(1,3);
keqaef(1) = (k23aef(1)*k21aef(1)/(x1(1)*k23aef(1)+(1-x1(1))*k21aef(1)));
equil = equilibrio(x1i(1),T(1));
P2vap(1) = equil(1,1);
gama2(1) = equil(1,2);
y2(1) = ((V(1)*y2b/dz)+param(10)*S*keqaef(1)*x2(1))/(((2*V(1)-Vb)/dz)+(param(10)*S*keqaef(1)*101.325/(P2vap(1)*gama2(1))));
H(1) = 36172.03-2919.83*y1(1)+(31.461-11.976*y1(1))*T(1)+(4.063e-4+0.0734*y1(1))*T(1)^2;


for i = 2:N
    Kaef = transf_masa2(x1(i),L(i),T(i),param);
    k13aef(i) = Kaef(1,1);
    V(i) = ((y1(i)*V(i-1)/dz)+param(10)*S*k13aef(i)*(x1(i)-x1i(i)))/((2*y1(i)-y1(i-1))/dz);
    k21aef(i) = Kaef(1,2);
    k23aef(i) = Kaef(1,3);
    keqaef(i) = (k23aef(i)*k21aef(i)/(x1(i)*k23aef(i)+(1-x1(i))*k21aef(i)));
    equil = equilibrio(x1i(i),T(i));
    P2vap(i) = equil(1,1);
    gama2(i) = equil(1,2);
    y2(i) = ((V(i)*y2(i-1)/dz)+param(10)*S*keqaef(i)*x2(i))/(((2*V(i)-V(i-1))/dz)+(param(10)*S*keqaef(i)*101.325/(P2vap(i)*gama2(i))));
    H(i) = 36172.03-2919.83*y1(i)+(31.461-11.976*y1(i))*T(i)+(4.063e-4+0.0734*y1(i))*T(i)^2;
end

    yD = polyval(coef_num_y_eq,x1c)/polyval(coef_den_y_eq,x1c);
    R = (yD-y1(N))/(y1(N)-x1c);                                              % [-]
    Lc = V(N)/(1+(1/R));                                             % [mol/s]
    Tc = (374.1+5855*x1c)/(1+16.65*x1c+0.1086*x1c^2);                    % [K]
    equil = equilibrio(x1c,Tc);                          % [Unidades varias]                               
    P2vap = equil(1,1);                                             % [kPa]                                                
    gama2 = equil(1,2);                                               % [-]
    x2c = V(N)*y2(N)/(Lc*(1+(P2vap*gama2/(101.325*R))));                    % [-]
    hc = (55.678*x1c+75.425)*Tc-15208.44*x1c-20602.34;              % [J/mol]

% Finalmente se presentan las ecuaciones diferenciales del modelo:
x_dot=zeros(4*N+No,1);

x_dot(1) = L(1)-Vb;
x_dot(2) = (1/Mb)*(L(1)*(x1(1)-x1b)-Vb*(y1b-x1b));
x_dot(3) = (1/Mb)*(L(1)*(x2(1)-x2b)-Vb*(y2b-x2b));
x_dot(4) = ((L(2)-L(1))/dz)+((Vb-V(1))/dz);
x_dot(5) = (1/M(1))*(L(1)*((x1(2)-x1(1))/dz)+V(1)*((y1b-y1(1))/dz)+(x1(1)-y1(1))*((V(1)-Vb)/dz));
x_dot(6) = (1/M(1))*(L(1)*((x2(2)-x2(1))/dz)+V(1)*((y2b-y2(1))/dz)+(x2(1)-y2(1))*((V(1)-Vb)/dz));
x_dot(7) = ((Mcp_c+mrp*cpr+M(1)*(55.678*x1(1)+75.425))^-1)*(-Q_loss/dz+L(1)*((h(2)-h(1))/dz)+V(1)*((Hb-H(1))/dz)+(h(1)-H(1))*((V(1)-Vb)/dz)-(55.678*T(1)-15208.44)*(L(1)*((x1(2)-x1(1))/dz)+V(1)*((y1b-y1(1))/dz)+(x1(1)-y1(1))*((V(1)-Vb)/dz)));
for i = 2:(N-1)
    x_dot(4*i) = ((L(i+1)-L(i))/dz)+((V(i-1)-V(i))/dz);
    x_dot(4*i+1) = (1/M(i))*(L(i)*((x1(i+1)-x1(i))/dz)+V(i)*((y1(i-1)-y1(i))/dz)+(x1(i)-y1(i))*((V(i)-V(i-1))/dz));
    x_dot(4*i+2) = (1/M(i))*(L(i)*((x2(i+1)-x2(i))/dz)+V(i)*((y2(i-1)-y2(i))/dz)+(x2(i)-y2(i))*((V(i)-V(i-1))/dz));
    x_dot(4*i+3) = ((Mcp_c+mrp*cpr+M(i)*(55.678*x1(i)+75.425))^-1)*(-Q_loss/dz+L(i)*((h(i+1)-h(i))/dz)+V(i)*((H(i-1)-H(i))/dz)+(h(i)-H(i))*((V(i)-V(i-1))/dz)-(55.678*T(i)-15208.44)*(L(i)*((x1(i+1)-x1(i))/dz)+V(i)*((y1(i-1)-y1(i))/dz)+(x1(i)-y1(i))*((V(i)-V(i-1))/dz)));
end
x_dot(4*N) = ((Lc-L(N))/dz)+((V(N-1)-V(N))/dz);
x_dot(4*N+1) = (1/M(N))*(L(N)*((x1c-x1(N))/dz)+V(N)*((y1(N-1)-y1(N))/dz)+(x1(N)-y1(N))*((V(N)-V(N-1))/dz));
x_dot(4*N+2) = (1/M(N))*(L(N)*((x2c-x2(N))/dz)+V(N)*((y2(N-1)-y2(N))/dz)+(x2(N)-y2(N))*((V(N)-V(N-1))/dz));
x_dot(4*N+3) = ((Mcp_c+mrp*cpr+M(N)*(55.678*x1(N)+75.425))^-1)*(-Q_loss/dz+L(N)*((hc-h(N))/dz)+V(N)*((H(N-1)-H(N))/dz)+(h(N)-H(N))*((V(N)-V(N-1))/dz)-(55.678*T(N)-15208.44)*(L(N)*((x1c-x1(N))/dz)+V(N)*((y1(N-1)-y1(N))/dz)+(x1(N)-y1(N))*((V(N)-V(N-1))/dz)));

% Se procede a calcular el volumen de destilado que es retirado del siste-
% ma:
destil = destilado(V(N),y1(N),y2(N),Lc,x1c,x2c,PM_EtOH,PM_H2O);
GL=destil(1,1);
Dvol=destil(1,2);
%     salida = [GL Dvol D_EtOH D_MEtOH D_H2O];  

x_dot(4*N+4) = destil(1,3);  %33  D_EtOH
x_dot(4*N+5) = destil(1,4);  %34  D_MEtOH
x_dot(4*N+6) = destil(1,5);  %34  D_H2O
x_dot(4*N+7)= (GL-GL_m)/(7.35/Dvol);    %40 Eq. dif sensor, cte tiempo: V/Dvol (seg)

N_et=x(4*N+4);
N_met=x(4*N+5);
N_w=x(4*N+6);

%% Output variables calculation
x1_ac=N_et/(N_et+N_met+N_w) ; % Ethanol mole fraction destilate drum
x2_ac=N_met/(N_et+N_met+N_w); % Methanol mole fraction distilate drum
dens_ac = densidad(x1_ac,293.15,PM_EtOH,PM_H2O); 
rho_1ac=dens_ac(1,2); % pure alcohol density in destialte drum
rho_13ac=dens_ac(1,3); % solution density in destialte drum
Mt=N_et*PM_EtOH+N_met*PM_MetOH+N_w*PM_H2O;
rho_methanol=0.789; % Density of pure methanol 20°C
Cmet=x2_ac*(1/rho_methanol)*1000;
GL_ac=x1_ac*(1/rho_1ac)*100/(1/rho_13ac);
Rec_eth=N_et*100/(x0(1)*x0(2));
Rec_met=N_met*100/(x0(1)*x0(3));

y=zeros(12,1);
y(1) = GL_m;   %35  GL
y(2)=GL;
y(3)=GL_ac;  %mL/s  Volumetric flow
y(4) =Tc;    %36  Tc
y(5) =Tb;    %37  
y(6) =x1c;   %38
y(7) =x2c;    %39
y(8)=Cmet;   %g/L a.a.
y(9)=Rec_eth;   %Ethanol molar flow mol/s
y(10)=Rec_met;   %Methanol molar flow mol/s
y(11)=Mt*rho_13ac/1000 ; % Destilate volumen  L
y(12)=Dvol; %mL/min Flow distillate
